simulink model "DDDR"  (R2020a)
settings: Solver=FixedStepAuto  StartTime=0.0  StopTime=50.0  FixedStep=1e-3  RelTol=1e-3  EnableMultiTasking=on
undefined symbols (not defined in the file): A0, A1, A3, D0, D1, D10, D11, D12, D13, D2, D3, D4, D5, D6, D7, D8, D9, PTA0, PTA1, PTA2, PTB11, PTB2, PTB23, PTB3, PTB9, PTC16, PTC17, PTC2, PTC3, PTC4, PTD0, PTD1, PTD2, PTD3
libraries: etargetslib x44, frdmk64flib x22, dspstat3 x1
(part 1 of 2)
settings Model: ExtModeTrigDuration=5  Creator=safanaal-emara  LastModifiedBy=prana
settings OptimizationCC: EnhancedBackFolding=on  PassReuseOutputArgsAs=Individual arguments  ZeroExternalMemoryAtStartup=off  ZeroInternalMemoryAtStartup=off  MaxStackSize=64  OptimizeBlockOrder=speed  DifferentSizesBufferReuse=on  OptimizationCustomize=off  EfficientTunableParamExpr=on
settings DebuggingCC: ParameterTunabilityLossMsg=error
settings HardwareCC: ProdBitPerPointer=32  ProdBitPerSizeT=32  ProdBitPerPtrDiffT=32  ProdLargestAtomicInteger=Long  ProdLargestAtomicFloat=Double  ProdWordSize=32  ProdHWDeviceType=ARM Compatible->ARM Cortex
settings SFSimCC: MATLABDynamicMemAlloc=off
settings RTWCC: SystemTargetFile=ert.tlc  HardwareBoard=NXP FRDM-K64F  TemplateMakefile=ert_default_tmf  Toolchain=GNU Tools for ARM Embedded Processors
settings CodeAppCC: ForceParamTrailComments=on  IgnoreCustomStorageClasses=off  OperatorAnnotations=on  SimulinkDataObjDesc=on  SFDataObjDesc=on  InsertBlockDesc=on
settings ERTTargetCC: SupportVariableSizeSignals=on

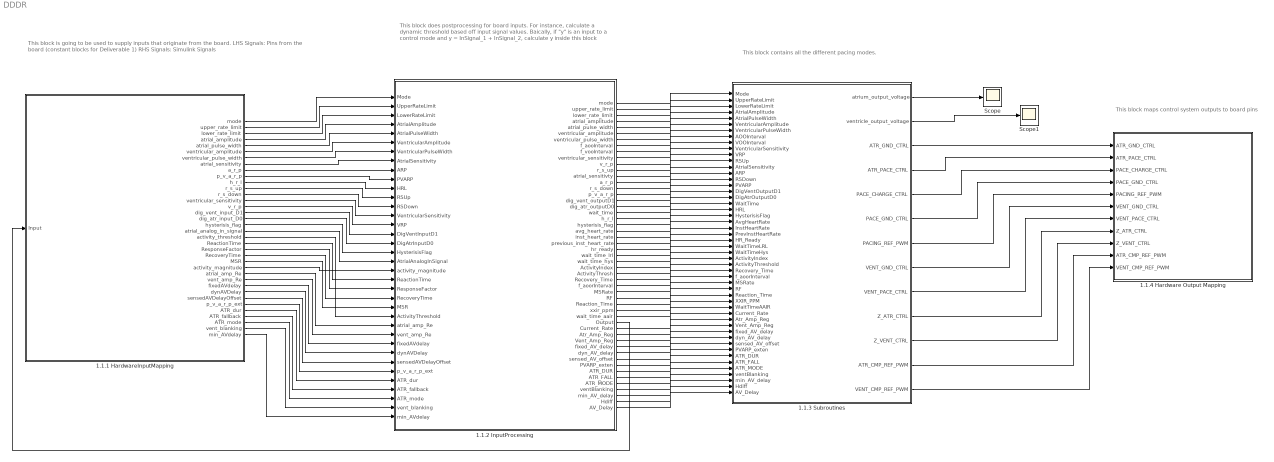
== system DDDR ==
  note: This block is going to be used to supply inputs that originate from the board.
      | LHS Signals: Pins from the board (constant blocks for Deliverable 1)
      | RHS Signals: Simulink Signals
  note: This block contains all the different pacing modes.
  note: This block does postprocessing for board inputs.
      | For instance, calculate a dynamic threshold based off input signal values.
      | Baically, if "y" is an input to a control mode and y = InSignal_1 + InSignal_2,
      | calculate y inside this block
  note: This block maps control system outputs to board pins
  1.1.1 HardwareInputMapping : Subsystem
  1.1.2 InputProcessing : Subsystem
  1.1.3 Subroutines : Subsystem
  1.1.4 Hardware Output Mapping : Subsystem
  Scope : Scope
  Scope1 : Scope
  wires:
  1.1.1 HardwareInputMapping/23(RecoveryTime) -> 1.1.2 InputProcessing/23(RecoveryTime)
  1.1.2 InputProcessing/30(Recovery_Time) -> 1.1.3 Subroutines/30(Recovery_Time)
  1.1.3 Subroutines/5(PACE_CHARGE_CTRL) -> 1.1.4 Hardware Output Mapping/3(PACE_CHARGE_CTRL)
  1.1.2 InputProcessing/31(f_aoorInterval) -> 1.1.3 Subroutines/31(f_aoorInterval)
  1.1.2 InputProcessing/19(wait_time) -> 1.1.3 Subroutines/19(WaitTime)
  1.1.2 InputProcessing/29(ActivityThresh) -> 1.1.3 Subroutines/29(ActivityThreshold)
  1.1.1 HardwareInputMapping/20(activity_threshold) -> 1.1.2 InputProcessing/25(ActivityThreshold)
  1.1.3 Subroutines/8(VENT_GND_CTRL) -> 1.1.4 Hardware Output Mapping/6(VENT_GND_CTRL)
  1.1.1 HardwareInputMapping/5(atrial_pulse_width) -> 1.1.2 InputProcessing/5(AtrialPulseWidth)
  1.1.3 Subroutines/12(ATR_CMP_REF_PWM) -> 1.1.4 Hardware Output Mapping/10(ATR_CMP_REF_PWM)
  1.1.3 Subroutines/13(VENT_CMP_REF_PWM) -> 1.1.4 Hardware Output Mapping/11(VENT_CMP_REF_PWM)
  1.1.2 InputProcessing/28(ActivityIndex) -> 1.1.3 Subroutines/28(ActivityIndex)
  1.1.3 Subroutines/6(PACE_GND_CTRL) -> 1.1.4 Hardware Output Mapping/4(PACE_GND_CTRL)
  1.1.2 InputProcessing/15(r_s_down) -> 1.1.3 Subroutines/15(RSDown)
  1.1.1 HardwareInputMapping/16(dig_vent_input_D1) -> 1.1.2 InputProcessing/16(DigVentInputD1)
  1.1.2 InputProcessing/32(MSRate) -> 1.1.3 Subroutines/32(MSRate)
  1.1.1 HardwareInputMapping/24(MSR) -> 1.1.2 InputProcessing/24(MSR)
  1.1.3 Subroutines/3(ATR_GND_CTRL) -> 1.1.4 Hardware Output Mapping/1(ATR_GND_CTRL)
  1.1.2 InputProcessing/26(wait_time_lrl) -> 1.1.3 Subroutines/26(WaitTimeLRL)
  1.1.2 InputProcessing/16(p_v_a_r_p) -> 1.1.3 Subroutines/16(PVARP)
  1.1.3 Subroutines/7(PACING_REF_PWM) -> 1.1.4 Hardware Output Mapping/5(PACING_REF_PWM)
  1.1.2 InputProcessing/27(wait_time_hys) -> 1.1.3 Subroutines/27(WaitTimeHys)
  1.1.2 InputProcessing/13(atrial_sensitivty) -> 1.1.3 Subroutines/13(AtrialSensitivity)
  1.1.2 InputProcessing/14(a_r_p) -> 1.1.3 Subroutines/14(ARP)
  1.1.1 HardwareInputMapping/3(lower_rate_limit) -> 1.1.2 InputProcessing/3(LowerRateLimit)
  1.1.2 InputProcessing/25(hr_ready) -> 1.1.3 Subroutines/25(HR_Ready)
  1.1.1 HardwareInputMapping/19(atrial_analog_in_signal) -> 1.1.2 InputProcessing/19(AtrialAnalogInSignal)
  1.1.2 InputProcessing/20(h_r_l) -> 1.1.3 Subroutines/20(HRL)
  1.1.2 InputProcessing/23(inst_heart_rate) -> 1.1.3 Subroutines/23(InstHeartRate)
  1.1.2 InputProcessing/10(ventricular_sensitivity) -> 1.1.3 Subroutines/10(VentricularSensitivity)
  1.1.2 InputProcessing/22(avg_heart_rate) -> 1.1.3 Subroutines/22(AvgHeartRate)
  1.1.3 Subroutines/11(Z_VENT_CTRL) -> 1.1.4 Hardware Output Mapping/9(Z_VENT_CTRL)
  1.1.3 Subroutines/10(Z_ATR_CTRL) -> 1.1.4 Hardware Output Mapping/8(Z_ATR_CTRL)
  1.1.3 Subroutines/9(VENT_PACE_CTRL) -> 1.1.4 Hardware Output Mapping/7(VENT_PACE_CTRL)
  1.1.1 HardwareInputMapping/14(ventricular_sensitivity) -> 1.1.2 InputProcessing/14(VentricularSensitivity)
  1.1.2 InputProcessing/34(Reaction_Time) -> 1.1.3 Subroutines/34(Reaction_Time)
  1.1.3 Subroutines/4(ATR_PACE_CTRL) -> 1.1.4 Hardware Output Mapping/2(ATR_PACE_CTRL)
  1.1.2 InputProcessing/17(dig_vent_outputD1) -> 1.1.3 Subroutines/17(DigVentOutputD1)
  1.1.1 HardwareInputMapping/11(h_r_l) -> 1.1.2 InputProcessing/11(HRL)
  1.1.1 HardwareInputMapping/7(ventricular_pulse_width) -> 1.1.2 InputProcessing/7(VentricularPulseWidth)
  1.1.1 HardwareInputMapping/10(p_v_a_r_p) -> 1.1.2 InputProcessing/10(PVARP)
  1.1.2 InputProcessing/11(v_r_p) -> 1.1.3 Subroutines/11(VRP)
  1.1.1 HardwareInputMapping/13(r_s_down) -> 1.1.2 InputProcessing/13(RSDown)
  1.1.2 InputProcessing/5(atrial_pulse_width) -> 1.1.3 Subroutines/5(AtrialPulseWidth)
  1.1.1 HardwareInputMapping/9(a_r_p) -> 1.1.2 InputProcessing/9(ARP)
  1.1.2 InputProcessing/36(wait_time_aair) -> 1.1.3 Subroutines/36(WaitTimeAAIR)
  1.1.2 InputProcessing/21(hysterisis_flag) -> 1.1.3 Subroutines/21(HysterisisFlag)
  1.1.1 HardwareInputMapping/17(dig_atr_input_D0) -> 1.1.2 InputProcessing/17(DigAtrInputD0)
  1.1.2 InputProcessing/7(ventricular_pulse_width) -> 1.1.3 Subroutines/7(VentricularPulseWidth)
  1.1.1 HardwareInputMapping/8(atrial_sensitivity) -> 1.1.2 InputProcessing/8(AtrialSensitivity)
  1.1.1 HardwareInputMapping/6(ventricular_amplitude) -> 1.1.2 InputProcessing/6(VentricularAmplitude)
  1.1.2 InputProcessing/33(RF) -> 1.1.3 Subroutines/33(RF)
  1.1.2 InputProcessing/3(lower_rate_limit) -> 1.1.3 Subroutines/3(LowerRateLimit)
  1.1.2 InputProcessing/24(previous_inst_heart_rate) -> 1.1.3 Subroutines/24(PrevInstHeartRate)
  1.1.2 InputProcessing/12(r_s_up) -> 1.1.3 Subroutines/12(RSUp)
  1.1.1 HardwareInputMapping/4(atrial_amplitude) -> 1.1.2 InputProcessing/4(AtrialAmplitude)
  1.1.2 InputProcessing/18(dig_atr_outputD0) -> 1.1.3 Subroutines/18(DigAtrOutputD0)
  1.1.3 Subroutines/2(ventricle_output_voltage) -> Scope1/1
  1.1.1 HardwareInputMapping/1(mode) -> 1.1.2 InputProcessing/1(Mode)
  1.1.3 Subroutines/1(atrium_output_voltage) -> Scope/1
  1.1.1 HardwareInputMapping/21(ReactionTime) -> 1.1.2 InputProcessing/21(ReactionTime)
  1.1.2 InputProcessing/4(atrial_amplitude) -> 1.1.3 Subroutines/4(AtrialAmplitude)
  1.1.2 InputProcessing/6(ventricular_amplitude) -> 1.1.3 Subroutines/6(VentricularAmplitude)
  1.1.1 HardwareInputMapping/18(hysterisis_flag) -> 1.1.2 InputProcessing/18(HysterisisFlag)
  1.1.2 InputProcessing/9(f_vooInterval) -> 1.1.3 Subroutines/9(VOOInterval)
  1.1.2 InputProcessing/1(mode) -> 1.1.3 Subroutines/1(Mode)
  1.1.1 HardwareInputMapping/22(ResponseFactor) -> 1.1.2 InputProcessing/22(ResponseFactor)
  1.1.1 HardwareInputMapping/15(v_r_p) -> 1.1.2 InputProcessing/15(VRP)
  1.1.1 HardwareInputMapping/2(upper_rate_limit) -> 1.1.2 InputProcessing/2(UpperRateLimit)
  1.1.2 InputProcessing/2(upper_rate_limit) -> 1.1.3 Subroutines/2(UpperRateLimit)
  1.1.1 HardwareInputMapping/12(r_s_up) -> 1.1.2 InputProcessing/12(RSUp)
  1.1.2 InputProcessing/8(f_aooInterval) -> 1.1.3 Subroutines/8(AOOInterval)
  1.1.2 InputProcessing/35(xxir_ppm) -> 1.1.3 Subroutines/35(XXIR_PPM)
  1.1.1 HardwareInputMapping/25(activity_magnitude) -> 1.1.2 InputProcessing/20(activity_magnitude)
  1.1.2 InputProcessing/37(Output) -> 1.1.1 HardwareInputMapping/1(Input)
  1.1.2 InputProcessing/38(Current_Rate) -> 1.1.3 Subroutines/37(Current_Rate)
  1.1.1 HardwareInputMapping/26(atrial_amp_Re) -> 1.1.2 InputProcessing/26(atrial_amp_Re)
  1.1.1 HardwareInputMapping/27(vent_amp_Re) -> 1.1.2 InputProcessing/27(vent_amp_Re)
  1.1.2 InputProcessing/39(Atr_Amp_Reg) -> 1.1.3 Subroutines/38(Atr_Amp_Reg)
  1.1.2 InputProcessing/40(Vent_Amp_Reg) -> 1.1.3 Subroutines/39(Vent_Amp_Reg)
  1.1.1 HardwareInputMapping/28(fixedAVdelay) -> 1.1.2 InputProcessing/28(fixedAVdelay)
  1.1.1 HardwareInputMapping/29(dynAVDelay) -> 1.1.2 InputProcessing/29(dynAVDelay)
  1.1.1 HardwareInputMapping/30(sensedAVDelayOffset) -> 1.1.2 InputProcessing/30(sensedAVDelayOffset)
  1.1.1 HardwareInputMapping/31(p_v_a_r_p_ext) -> 1.1.2 InputProcessing/31(p_v_a_r_p_ext)
  1.1.1 HardwareInputMapping/32(ATR_dur) -> 1.1.2 InputProcessing/32(ATR_dur)
  1.1.1 HardwareInputMapping/33(ATR_fallback) -> 1.1.2 InputProcessing/33(ATR_fallback)
  1.1.1 HardwareInputMapping/34(ATR_mode) -> 1.1.2 InputProcessing/34(ATR_mode)
  1.1.1 HardwareInputMapping/35(vent_blanking) -> 1.1.2 InputProcessing/35(vent_blanking)
  1.1.1 HardwareInputMapping/36(min_AVdelay) -> 1.1.2 InputProcessing/36(min_AVdelay)
  1.1.2 InputProcessing/41(fixed_AV_delay) -> 1.1.3 Subroutines/40(fixed_AV_delay)
  1.1.2 InputProcessing/42(dyn_AV_delay) -> 1.1.3 Subroutines/41(dyn_AV_delay)
  1.1.2 InputProcessing/43(sensed_AV_offset) -> 1.1.3 Subroutines/42(sensed_AV_offset)
  1.1.2 InputProcessing/44(PVARP_exten) -> 1.1.3 Subroutines/43(PVARP_exten)
  1.1.2 InputProcessing/45(ATR_DUR) -> 1.1.3 Subroutines/44(ATR_DUR)
  1.1.2 InputProcessing/46(ATR_FALL) -> 1.1.3 Subroutines/45(ATR_FALL)
  1.1.2 InputProcessing/47(ATR_MODE) -> 1.1.3 Subroutines/46(ATR_MODE)
  1.1.2 InputProcessing/48(ventBlanking) -> 1.1.3 Subroutines/47(ventBlanking)
  1.1.2 InputProcessing/49(min_AV_delay) -> 1.1.3 Subroutines/48(min_AV_delay)
  1.1.2 InputProcessing/50(Hdiff) -> 1.1.3 Subroutines/49(Hdiff)
  1.1.2 InputProcessing/51(AV_Delay) -> 1.1.3 Subroutines/50(AV_Delay)

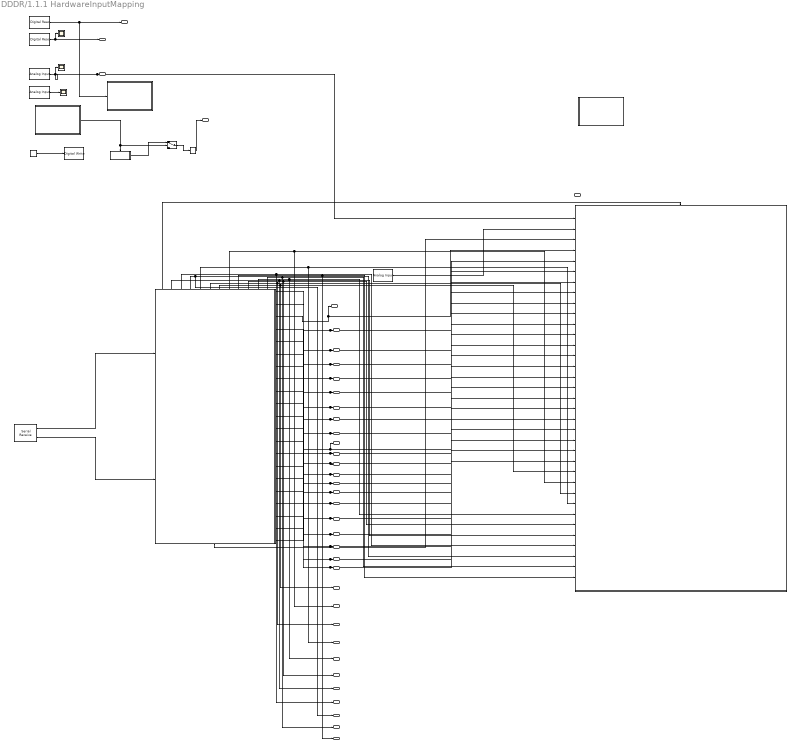
== system DDDR/1.1.1 HardwareInputMapping ==
  note: Technically should be in 1.1.2, but remains here for sake of testing ease
  note: Hardware Abstraction
  Input : Inport  OutDataTypeStr=uint32
  ATR_CMP_DETECT : frdmk64flib/Digital Read  Whichpin=PTC16 (D0)  SampleTime=0.001
  Analog Input : frdmk64flib/Analog Input  Whichpin=PTB2 (A0)  SampleTime=0.001
  Analog Input1 : frdmk64flib/Analog Input  Whichpin=PTB11 (A3)  SampleTime=0.001
  Analog Input4 : frdmk64flib/Analog Input  Whichpin=PTB3 (A1)  SampleTime=0.001
  Chart1 : Stateflow chart  TreatAsAtomicUnit=on
      settings: PortSchema="{\"entries\":[{\"content\":{\"sides\":[{\"content\":{\"connectorIds\":[\"In1\",\"In2\"]},\"type\":\"ConnectorPlacement.EquallySpacedRectSide\",\"uuid\":\"4b4e7b92-92d9-42ab-8219-d0bebd29739c\"},{\"content\":{\"connectorIds\":[\"Out2\",\"Out3\",\"Out4\",\"Out5\",\"Out6\",\"Out7\",\"Out8\",\"Out9\",\"Out10\",\"Out11\",\"Out12\",\"Out13\",\"Out14\",\"Out15\",\"Out16\",\"Out17\",\"Out18\",\"Out19\",\"Out20\",\"Out21\",\"Out22\"],\"side\":\"RIGHT\"},\"type\":\"ConnectorPlacement.EquallySpacedRectSide\",\"uuid\":\"63818af1-55be-4bb8-9c31-e72eb1b14a30\"},{\"content\":{\"connectorIds\":[\"Out23\",\"Out24\",\"Out25\",\"Out26\",\"Out27\",\"Out28\",\"Out29\",\"Out30\",\"Out31\",\"Out32\",\"Out33\",\"Out34\"],\"side\":\"TOP\"},\"type\":\"ConnectorPlacement.EquallySpacedRectSide\",\"uuid\":\"fba88a00-7af7-4cc1-9c88-2f6823948803\"},{\"content\":{\"connectorIds\":[\"Out1\"],\"side\":\"BOTTOM\"},\"type\":\"ConnectorPlacement.EquallySpacedRectSide\",\"uuid\":\"45b0438b-424b-4dc6-9f15-00cd0d7c78e5\"}]},\"type\":\"ConnectorPlacement.EquallySpacedConnector\",\"uuid\":\"faeef76d-5f3a-4672-ae10-d5c9531e9562\"}],\"packageUris\":[\"http://schema.mathworks.com/mf0/Connector/19700101\"],\"version\":\"1.0\"}"
  Constant15 : Constant  Value=true  OutDataTypeStr=boolean
  Digital Write1 : frdmk64flib/Digital Write  Whichpin=PTD1 (D13)
  HeartChamberPulseDetection : Stateflow chart  TreatAsAtomicUnit=on
  HeartChamberPulseDetection2 : Stateflow chart  TreatAsAtomicUnit=on
  HeartChamberPulseDetection3 : Stateflow chart  TreatAsAtomicUnit=on
  Memory : Memory
  Scope : Scope
  Scope1 : Scope
  Scope2 : Scope
  Serial Receive : frdmk64flib/Serial Receive  SCIModule=0  Baudrate=uint32(9600)  Parity=None  StopBits=1  HardwareFlowControl=None  ByteOrder=LittleEndian  DataType=uint8  DataLength=125  BlockingMode=off  OutputStatus=on  SampleTime=-1
  Subsystem1 : Subsystem
  Switch : Switch  Criteria=u2 > Threshold
  Triggered Subsystem : Subsystem  TreatAsAtomicUnit=on
  VENT_CMP_DETECT : frdmk64flib/Digital Read  Whichpin=PTC17 (D1)  SampleTime=0.001
  mode : Outport  OutDataTypeStr=uint32
  upper_rate_limit : Outport  Port=2
  lower_rate_limit : Outport  Port=3  OutDataTypeStr=uint32
  atrial_amplitude : Outport  Port=4
  atrial_pulse_width : Outport  Port=5
  ventricular_amplitude : Outport  Port=6
  ventricular_pulse_width : Outport  Port=7
  atrial_sensitivity : Outport  Port=8
  a_r_p : Outport  Port=9
  p_v_a_r_p : Outport  Port=10
  h_r_l : Outport  Port=11
  r_s_up : Outport  Port=12
  r_s_down : Outport  Port=13
  ventricular_sensitivity : Outport  Port=14
  v_r_p : Outport  Port=15
  dig_vent_input_D1 : Outport  Port=16
  dig_atr_input_D0 : Outport  Port=17
  hysterisis_flag : Outport  Port=18
  atrial_analog_in_signal : Outport  Port=19
  activity_threshold : Outport  Port=20
  ReactionTime : Outport  Port=21
  ResponseFactor : Outport  Port=22
  RecoveryTime : Outport  Port=23
  MSR : Outport  Port=24
  activity_magnitude : Outport  Port=25
  atrial_amp_Re : Outport  Port=26
  vent_amp_Re : Outport  Port=27
  fixedAVdelay : Outport  Port=28
  dynAVDelay : Outport  Port=29
  sensedAVDelayOffset : Outport  Port=30
  p_v_a_r_p_ext : Outport  Port=31
  ATR_dur : Outport  Port=32
  ATR_fallback : Outport  Port=33
  ATR_mode : Outport  Port=34
  vent_blanking : Outport  Port=35
  min_AVdelay : Outport  Port=36
  wires:
  ATR_CMP_DETECT/1 -> Scope/1, dig_atr_input_D0/1
  Constant15/1 -> Digital Write1/1
  VENT_CMP_DETECT/1 -> dig_vent_input_D1/1, HeartChamberPulseDetection/1(in_voltage)
  Chart1/4(Mode) -> Subsystem1/4(Mode), mode/1
  Chart1/2(MSR) -> Subsystem1/24(m_s_r), MSR/1
  Chart1/3(ReactionTime) -> Subsystem1/21(Reaction_time), ReactionTime/1
  Chart1/5(RecoveryTime) -> Subsystem1/23(recovery_time), RecoveryTime/1
  Chart1/6(ResponseFactor) -> Subsystem1/22(Response_factor), ResponseFactor/1
  Chart1/7(a_r_p) -> Subsystem1/12(ARP), a_r_p/1
  Chart1/9(atrial_amplitude) -> Subsystem1/7(AtrialAmplitude), atrial_amplitude/1
  Chart1/10(atrial_pulse_width) -> Subsystem1/8(AtrialPulseWidth), atrial_pulse_width/1
  Chart1/11(atrial_sensitivity) -> Subsystem1/11(AtrialSensitivity), atrial_sensitivity/1
  Chart1/12(h_r_l) -> Subsystem1/14(HRL), h_r_l/1
  Chart1/13(hysterisis_flag) -> Subsystem1/18(HysterisisFlag1), hysterisis_flag/1
  Chart1/14(lower_rate_limit) -> Subsystem1/6(LowerRateLimit), lower_rate_limit/1
  Chart1/15(p_v_a_r_p) -> Subsystem1/13(PVARP), p_v_a_r_p/1
  Chart1/16(r_s_down) -> Subsystem1/16(RSDown), r_s_down/1
  Chart1/17(r_s_up) -> Subsystem1/15(RSUp), r_s_up/1
  Chart1/18(upper_rate_limit) -> Subsystem1/5(UpperRateLimit), upper_rate_limit/1
  Chart1/19(v_r_p) -> Subsystem1/19(VRP), v_r_p/1
  Chart1/20(ventricular_amplitude) -> Subsystem1/9(VentricularAmplitude), ventricular_amplitude/1
  Chart1/21(ventricular_pulse_width) -> Subsystem1/10(VentricularPulseWidth), ventricular_pulse_width/1
  Chart1/22(ventricular_sensitivity) -> Subsystem1/17(VentricularSensitivity), ventricular_sensitivity/1
  Serial Receive/1 -> Chart1/1(rx_data)
  Serial Receive/2 -> Chart1/2(status)
  Chart1/23(MSG_trigger) -> Subsystem1/Trigger
  Chart1/8(activity_threshold) -> Subsystem1/20(Activity_threshold), activity_threshold/1
  HeartChamberPulseDetection3/1(LED_STATE) -> Triggered Subsystem/Trigger, Switch/2
  Switch/1 -> Memory/1
  Memory/1 -> activity_magnitude/1
  Triggered Subsystem/1(activity_magnitude) -> Switch/1
  Chart1/1(MSG_ident) -> Subsystem1/3(MSG_ident)
  Analog Input4/1 -> Subsystem1/2(Vent_signal)
  Analog Input1/1 -> Scope2/1
  Analog Input/1 -> Subsystem1/1(Atrial_signal), atrial_analog_in_signal/1, Scope1/1
  Chart1/29(atrial_amplitude_Re) -> atrial_amp_Re/1, Subsystem1/25(atr_amp_re)
  Chart1/30(ventricular_amplitude_Re) -> vent_amp_Re/1, Subsystem1/26(vent_amp_re)
  Chart1/28(Fixed_AV_delay) -> fixedAVdelay/1, Subsystem1/27(fixed_AV_delay)
  Chart1/27(Dynamic_AV_delay) -> dynAVDelay/1, Subsystem1/28(dynamic_AV_delay)
  Chart1/33(sensed_AV_delay_offset) -> sensedAVDelayOffset/1, Subsystem1/29(sensed_AV_delay_offset)
  Chart1/32(p_v_a_r_p_ext) -> p_v_a_r_p_ext/1, Subsystem1/30(pvarp_ext)
  Chart1/24(ATR_dur) -> ATR_dur/1, Subsystem1/31(ATR_dur)
  Chart1/25(ATR_fallback_time) -> ATR_fallback/1, Subsystem1/32(ATR_fallback)
  Chart1/26(ATR_mode) -> ATR_mode/1, Subsystem1/33(ATR_mode)
  Chart1/34(vent_blanking) -> vent_blanking/1, Subsystem1/34(vent_blanking)
  Chart1/31(min_AV_delay) -> min_AVdelay/1, Subsystem1/35(min_dyn_AV_delay)

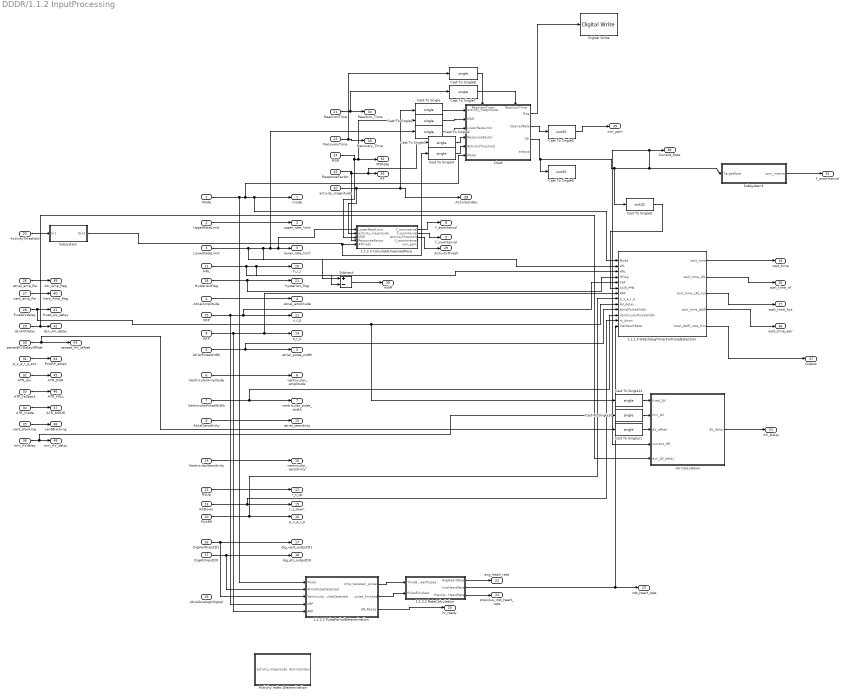
== system DDDR/1.1.2 InputProcessing ==
  Mode : Inport
  UpperRateLimit : Inport  Port=2
  LowerRateLimit : Inport  Port=3  OutDataTypeStr=uint32
  AtrialAmplitude : Inport  Port=4
  AtrialPulseWidth : Inport  Port=5
  VentricularAmplitude : Inport  Port=6
  VentricularPulseWidth : Inport  Port=7
  AtrialSensitivity : Inport  Port=8
  ARP : Inport  Port=9
  PVARP : Inport  Port=10
  HRL : Inport  Port=11
  RSUp : Inport  Port=12
  RSDown : Inport  Port=13
  VentricularSensitivity : Inport  Port=14
  VRP : Inport  Port=15
  DigVentInputD1 : Inport  Port=16
  DigAtrInputD0 : Inport  Port=17
  HysterisisFlag : Inport  Port=18
  AtrialAnalogInSignal : Inport  Port=19
  activity_magnitude : Inport  Port=20
  ReactionTime : Inport  Port=21
  ResponseFactor : Inport  Port=22
  RecoveryTime : Inport  Port=23
  MSR : Inport  Port=24
  ActivityThreshold : Inport  Port=25
  atrial_amp_Re : Inport  Port=26
  vent_amp_Re : Inport  Port=27
  fixedAVdelay : Inport  Port=28
  dynAVDelay : Inport  Port=29
  sensedAVDelayOffset : Inport  Port=30
  p_v_a_r_p_ext : Inport  Port=31
  ATR_dur : Inport  Port=32
  ATR_fallback : Inport  Port=33
  ATR_mode : Inport  Port=34
  vent_blanking : Inport  Port=35
  min_AVdelay : Inport  Port=36
  1.1.2.1 PulsePeriodDetermination : Stateflow chart  TreatAsAtomicUnit=on
  1.1.2.2 RateCalculation : Subsystem
  1.1.2.3 WatchdogTimerForPulseDetection : Stateflow chart  TreatAsAtomicUnit=on
      settings: PortSchema="{\"entries\":[{\"content\":{\"sides\":[{\"content\":{\"connectorIds\":[\"In2\",\"In4\",\"In3\",\"In1\",\"In8\",\"In10\",\"In11\",\"In12\",\"In13\",\"In5\",\"In6\",\"In9\",\"In7\"]},\"type\":\"ConnectorPlacement.EquallySpacedRectSide\",\"uuid\":\"bdcd44c7-b2d4-4456-b1dc-ebe8b4250225\"},{\"content\":{\"connectorIds\":[\"Out1\",\"Out2\",\"Out3\",\"Out4\",\"Out5\"],\"side\":\"RIGHT\"},\"type\":\"ConnectorPlacement.EquallySpacedRectSide\",\"uuid\":\"3cd61675-91fc-4dc9-8435-a65c8d2417e3\"},{\"content\":{\"connectorIds\":[],\"side\":\"TOP\"},\"type\":\"ConnectorPlacement.EquallySpacedRectSide\",\"uuid\":\"27150ff9-b670-45e1-a88f-5aa1ecaf40ee\"}]},\"type\":\"ConnectorPlacement.EquallySpacedConnector\",\"uuid\":\"8013b024-43b4-4f43-9604-3ddd237ba5b0\"}],\"packageUris\":[\"http://schema.mathworks.com/mf0/Connector/19700101\"],\"version\":\"1.0\"}"
  1.1.2.4 CalculateUnsensedPace : Subsystem
  AV Calculation : Stateflow chart  TreatAsAtomicUnit=on
  Activity Index Determination : Stateflow chart  TreatAsAtomicUnit=on
  Cast To Single{,1..4,7..8,10..12} (10 alike) : DataTypeConversion  OutDataTypeStr=single
  Cast To Single5 : DataTypeConversion  OutDataTypeStr=uint32
  Cast To Single6 : DataTypeConversion  OutDataTypeStr=uint32
  Cast To Single9 : DataTypeConversion  OutDataTypeStr=uint32
  Chart : Stateflow chart  TreatAsAtomicUnit=on
      settings: PortSchema="{\"entries\":[{\"content\":{\"sides\":[{\"content\":{\"connectorIds\":[\"In3\",\"In4\",\"In5\",\"In6\",\"In7\",\"In8\"]},\"type\":\"ConnectorPlacement.EquallySpacedRectSide\",\"uuid\":\"2448e127-c765-4c5f-8f36-5c1cc0db25c5\"},{\"content\":{\"connectorIds\":[\"Out1\",\"Out2\",\"Out3\",\"Out4\"],\"side\":\"RIGHT\"},\"type\":\"ConnectorPlacement.EquallySpacedRectSide\",\"uuid\":\"7735dab6-aae1-403a-9bfd-50f09b6b5fda\"},{\"content\":{\"connectorIds\":[\"In1\",\"In2\"],\"side\":\"TOP\"},\"type\":\"ConnectorPlacement.EquallySpacedRectSide\",\"uuid\":\"b73b27d3-29c6-41fa-95b7-891e2a296021\"}]},\"type\":\"ConnectorPlacement.EquallySpacedConnector\",\"uuid\":\"e62d7f02-cd80-41b6-aa16-da75d3dcce48\"}],\"packageUris\":[\"http://schema.mathworks.com/mf0/Connector/19700101\"],\"version\":\"1.0\"}"
  Digital Write : frdmk64flib/Digital Write  Whichpin=GREEN_LED
  Subsystem : Subsystem
  Subsystem1 : Subsystem
  Subtract : Sum  Inputs=+-
  mode : Outport  OutDataTypeStr=uint32
  upper_rate_limit : Outport  Port=2
  lower_rate_limit : Outport  Port=3
  atrial_amplitude : Outport  Port=4
  atrial_pulse_width : Outport  Port=5
  ventricular_amplitude : Outport  Port=6
  ventricular_pulse_width : Outport  Port=7
  f_aooInterval : Outport  Port=8
  f_vooInterval : Outport  Port=9
  ventricular_sensitivity : Outport  Port=10
  v_r_p : Outport  Port=11
  r_s_up : Outport  Port=12
  atrial_sensitivty : Outport  Port=13
  a_r_p : Outport  Port=14
  r_s_down : Outport  Port=15
  p_v_a_r_p : Outport  Port=16
  dig_vent_outputD1 : Outport  Port=17
  dig_atr_outputD0 : Outport  Port=18
  wait_time : Outport  Port=19
  h_r_l : Outport  Port=20
  hysterisis_flag : Outport  Port=21
  avg_heart_rate : Outport  Port=22
  inst_heart_rate : Outport  Port=23
  previous_inst_heart_rate : Outport  Port=24
  hr_ready : Outport  Port=25
  wait_time_lrl : Outport  Port=26
  wait_time_hys : Outport  Port=27
  ActivityIndex : Outport  Port=28
  ActivityThresh : Outport  Port=29
  Recovery_Time : Outport  Port=30
  f_aoorInterval : Outport  Port=31  OutDataTypeStr=uint32
  MSRate : Outport  Port=32
  RF : Outport  Port=33
  Reaction_Time : Outport  Port=34
  xxir_ppm : Outport  Port=35
  wait_time_aair : Outport  Port=36
  Output : Outport  Port=37
  Current_Rate : Outport  Port=38
  Atr_Amp_Reg : Outport  Port=39
  Vent_Amp_Reg : Outport  Port=40
  fixed_AV_delay : Outport  Port=41
  dyn_AV_delay : Outport  Port=42
  sensed_AV_offset : Outport  Port=43
  PVARP_exten : Outport  Port=44
  ATR_DUR : Outport  Port=45
  ATR_FALL : Outport  Port=46
  ATR_MODE : Outport  Port=47
  ventBlanking : Outport  Port=48
  min_AV_delay : Outport  Port=49
  Hdiff : Outport  Port=50
  AV_Delay : Outport  Port=51  OutDataTypeStr=single
  wires:
  Mode/1 -> 1.1.2.1 PulsePeriodDetermination/1(Mode), Chart/8(Mode), 1.1.2.3 WatchdogTimerForPulseDetection/2(Mode), mode/1
  UpperRateLimit/1 -> upper_rate_limit/1
  LowerRateLimit/1 -> Subtract/1, Cast To Single2/1, 1.1.2.4 CalculateUnsensedPace/1(LowerRateLimit), lower_rate_limit/1, 1.1.2.3 WatchdogTimerForPulseDetection/4(LRL)
  AtrialAmplitude/1 -> atrial_amplitude/1
  AtrialPulseWidth/1 -> 1.1.2.3 WatchdogTimerForPulseDetection/5(AtrialPulseWidth), atrial_pulse_width/1
  VentricularAmplitude/1 -> ventricular_amplitude/1
  VentricularPulseWidth/1 -> 1.1.2.3 WatchdogTimerForPulseDetection/6(VentricularPulseWidth), ventricular_pulse_width/1
  1.1.2.4 CalculateUnsensedPace/1(f_aooInterval) -> f_aooInterval/1
  1.1.2.4 CalculateUnsensedPace/2(f_vooInterval) -> f_vooInterval/1
  VentricularSensitivity/1 -> ventricular_sensitivity/1
  VRP/1 -> 1.1.2.1 PulsePeriodDetermination/4(VRP), 1.1.2.3 WatchdogTimerForPulseDetection/8(VRP), v_r_p/1
  RSUp/1 -> r_s_up/1
  AtrialSensitivity/1 -> atrial_sensitivty/1
  ARP/1 -> 1.1.2.1 PulsePeriodDetermination/5(ARP), 1.1.2.3 WatchdogTimerForPulseDetection/11(ARP), a_r_p/1
  RSDown/1 -> 1.1.2.3 WatchdogTimerForPulseDetection/9(rs_down), r_s_down/1
  PVARP/1 -> 1.1.2.3 WatchdogTimerForPulseDetection/12(p_v_a_r_p), p_v_a_r_p/1
  HRL/1 -> Subtract/2, 1.1.2.3 WatchdogTimerForPulseDetection/3(HRL), h_r_l/1
  DigVentInputD1/1 -> 1.1.2.1 PulsePeriodDetermination/3(VentricularPulseDetected), dig_vent_outputD1/1
  DigAtrInputD0/1 -> 1.1.2.1 PulsePeriodDetermination/2(AtrialPulseDetected), dig_atr_outputD0/1
  HysterisisFlag/1 -> 1.1.2.3 WatchdogTimerForPulseDetection/1(HFlag), hysterisis_flag/1
  1.1.2.3 WatchdogTimerForPulseDetection/1(wait_time) -> wait_time/1
  1.1.2.1 PulsePeriodDetermination/1(time_between_pulses) -> 1.1.2.2 RateCalculation/1(TimeBetweenPulses)
  1.1.2.2 RateCalculation/1(AvgHeartRate) -> avg_heart_rate/1
  1.1.2.2 RateCalculation/3(PrevInstHeartRate) -> previous_inst_heart_rate/1
  1.1.2.2 RateCalculation/2(InstHeartRate) -> 1.1.2.3 WatchdogTimerForPulseDetection/7(InstHeartRate), inst_heart_rate/1
  1.1.2.1 PulsePeriodDetermination/3(HR_Ready) -> hr_ready/1
  1.1.2.1 PulsePeriodDetermination/2(pulse_finished) -> 1.1.2.2 RateCalculation/2(PulseFinished)
  1.1.2.3 WatchdogTimerForPulseDetection/2(wait_time_LRL) -> wait_time_lrl/1
  1.1.2.3 WatchdogTimerForPulseDetection/3(wait_time_LRL_hys) -> wait_time_hys/1
  activity_magnitude/1 -> 1.1.2.4 CalculateUnsensedPace/2(activity_magnitude), Cast To Single/1, ActivityIndex/1
  ActivityThreshold/1 -> Subsystem/1(In1)
  1.1.2.4 CalculateUnsensedPace/3(ActivityThreshold) -> ActivityThresh/1
  MSR/1 -> 1.1.2.4 CalculateUnsensedPace/3(MSR), MSRate/1, Cast To Single1/1
  ResponseFactor/1 -> Cast To Single3/1, RF/1, 1.1.2.4 CalculateUnsensedPace/4(ResponseFactor)
  RecoveryTime/1 -> Cast To Single8/1, Recovery_Time/1
  1.1.2.3 WatchdogTimerForPulseDetection/4(wait_time_AAIR) -> wait_time_aair/1
  Chart/1(flag) -> Digital Write/1
  Chart/2(DesiredRate) -> Cast To Single5/1
  Subsystem1/1(xoor_interval) -> f_aoorInterval/1
  Cast To Single/1 -> Chart/3(activity_magnitude)
  Cast To Single1/1 -> Chart/4(MSR)
  Cast To Single2/1 -> Chart/5(LowerRateLimit)
  Cast To Single3/1 -> Chart/6(ResponseFactor)
  Cast To Single4/1 -> Chart/7(ActivityThreshold)
  Cast To Single5/1 -> xxir_ppm/1
  ReactionTime/1 -> Cast To Single7/1, Reaction_Time/1
  Cast To Single8/1 -> Chart/1(RecoveryTime)
  Cast To Single7/1 -> Chart/2(ReactionTime)
  Chart/3(CR) -> Cast To Single6/1, Cast To Single9/1, Current_Rate/1, AV Calculation/4(current_HR), Subsystem1/1(TargetRate)
  Cast To Single9/1 -> 1.1.2.3 WatchdogTimerForPulseDetection/10(XXIR_PPM)
  1.1.2.3 WatchdogTimerForPulseDetection/5(total_AAIR_rate_time) -> Output/1
  Subsystem/1(Out1) -> Cast To Single4/1, 1.1.2.4 CalculateUnsensedPace/5(AThresh)
  atrial_amp_Re/1 -> Atr_Amp_Reg/1
  vent_amp_Re/1 -> Vent_Amp_Reg/1
  dynAVDelay/1 -> AV Calculation/5(dyn_AV_delay), dyn_AV_delay/1
  fixedAVdelay/1 -> Cast To Single12/1, 1.1.2.3 WatchdogTimerForPulseDetection/13(AV_delay), fixed_AV_delay/1
  p_v_a_r_p_ext/1 -> PVARP_exten/1
  sensedAVDelayOffset/1 -> Cast To Single11/1, sensed_AV_offset/1
  ATR_dur/1 -> ATR_DUR/1
  ATR_fallback/1 -> ATR_FALL/1
  ATR_mode/1 -> ATR_MODE/1
  vent_blanking/1 -> ventBlanking/1
  min_AVdelay/1 -> Cast To Single10/1, min_AV_delay/1
  Subtract/1 -> Hdiff/1
  AV Calculation/1(AV_delay) -> AV_Delay/1
  Cast To Single10/1 -> AV Calculation/2(min_AV)
  Cast To Single11/1 -> AV Calculation/3(AV_offset)
  Cast To Single12/1 -> AV Calculation/1(fixed_AV)

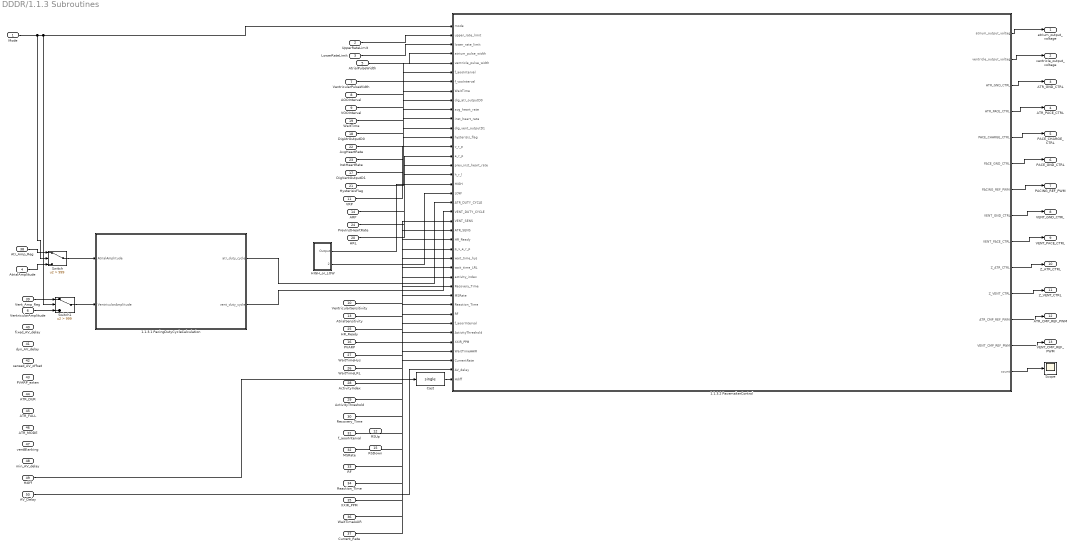
== system DDDR/1.1.3 Subroutines ==
  Mode : Inport
  UpperRateLimit : Inport  Port=2
  LowerRateLimit : Inport  Port=3
  AtrialAmplitude : Inport  Port=4
  AtrialPulseWidth : Inport  Port=5  OutDataTypeStr=double
  VentricularAmplitude : Inport  Port=6
  VentricularPulseWidth : Inport  Port=7  OutDataTypeStr=double
  AOOInterval : Inport  Port=8
  VOOInterval : Inport  Port=9
  VentricularSensitivity : Inport  Port=10
  VRP : Inport  Port=11
  RSUp : Inport  Port=12
  AtrialSensitivity : Inport  Port=13
  ARP : Inport  Port=14
  RSDown : Inport  Port=15
  PVARP : Inport  Port=16
  DigVentOutputD1 : Inport  Port=17
  DigAtrOutputD0 : Inport  Port=18
  WaitTime : Inport  Port=19
  HRL : Inport  Port=20
  HysterisisFlag : Inport  Port=21
  AvgHeartRate : Inport  Port=22
  InstHeartRate : Inport  Port=23
  PrevInstHeartRate : Inport  Port=24
  HR_Ready : Inport  Port=25
  WaitTimeLRL : Inport  Port=26
  WaitTimeHys : Inport  Port=27
  ActivityIndex : Inport  Port=28
  ActivityThreshold : Inport  Port=29
  Recovery_Time : Inport  Port=30
  f_aoorInterval : Inport  Port=31
  MSRate : Inport  Port=32
  RF : Inport  Port=33
  Reaction_Time : Inport  Port=34
  XXIR_PPM : Inport  Port=35
  WaitTimeAAIR : Inport  Port=36
  Current_Rate : Inport  Port=37
  Atr_Amp_Reg : Inport  Port=38
  Vent_Amp_Reg : Inport  Port=39
  fixed_AV_delay : Inport  Port=40
  dyn_AV_delay : Inport  Port=41
  sensed_AV_offset : Inport  Port=42
  PVARP_exten : Inport  Port=43
  ATR_DUR : Inport  Port=44
  ATR_FALL : Inport  Port=45
  ATR_MODE : Inport  Port=46
  ventBlanking : Inport  Port=47
  min_AV_delay : Inport  Port=48
  Hdiff : Inport  Port=49
  AV_Delay : Inport  Port=50
  1.1.3.1 PacingDutyCycleCalculation : Subsystem
  1.1.3.2 PacemakerControl : Stateflow chart  TreatAsAtomicUnit=on
      settings: PortSchema="{\"entries\":[{\"content\":{\"sides\":[{\"content\":{\"connectorIds\":[\"In1\",\"In2\",\"In3\",\"In4\",\"In5\",\"In6\",\"In7\",\"In8\",\"In12\",\"In10\",\"In11\",\"In9\",\"In13\",\"In14\",\"In15\",\"In16\",\"In17\",\"In18\",\"In19\",\"In20\",\"In21\",\"In22\",\"In23\",\"In24\",\"In25\",\"In26\",\"In27\",\"In28\",\"In29\",\"In30\",\"In31\",\"In32\",\"In33\",\"In34\",\"In35\",\"In36\",\"In37\",\"In38\",\"In39\"]},\"type\":\"ConnectorPlacement.EquallySpacedRectSide\",\"uuid\":\"d7a0a1d4-1adb-4f49-9409-b65f2a410999\"},{\"content\":{\"connectorIds\":[\"Out1\",\"Out2\",\"Out3\",\"Out4\",\"Out5\",\"Out6\",\"Out7\",\"Out8\",\"Out9\",\"Out10\",\"Out11\",\"Out12\",\"Out13\",\"Out14\"],\"side\":\"RIGHT\"},\"type\":\"ConnectorPlacement.EquallySpacedRectSide\",\"uuid\":\"f178eaad-70cd-4ec4-a78d-12af1cfbe493\"},{\"content\":{\"connectorIds\":[],\"side\":\"TOP\"},\"type\":\"ConnectorPlacement.EquallySpacedRectSide\",\"uuid\":\"df2c6513-3872-482b-abe5-5bf3da958119\"}]},\"type\":\"ConnectorPlacement.EquallySpacedConnector\",\"uuid\":\"0d6dffcb-0af9-47c5-9cde-377e88cba9d4\"}],\"packageUris\":[\"http://schema.mathworks.com/mf0/Connector/19700101\"],\"version\":\"1.0\"}"
  Cast : DataTypeConversion  OutDataTypeStr=single
  HIGH_or_LOW : Subsystem
      settings: PortSchema="{\"entries\":[{\"content\":{\"sides\":[{\"content\":{},\"type\":\"ConnectorPlacement.EquallySpacedRectSide\",\"uuid\":\"49d8c1b3-c71d-4c5e-9f29-3a8fe0514842\"},{\"content\":{\"side\":\"RIGHT\"},\"type\":\"ConnectorPlacement.EquallySpacedRectSide\",\"uuid\":\"0963f443-37bf-457e-bfcb-1d561403e5a9\"},{\"content\":{\"connectorIds\":[\"Out1\",\"Out2\"],\"side\":\"TOP\"},\"type\":\"ConnectorPlacement.EquallySpacedRectSide\",\"uuid\":\"32b78edd-16d0-4f55-b401-e4c12abc873e\"}]},\"type\":\"ConnectorPlacement.EquallySpacedConnector\",\"uuid\":\"974eb872-d95b-4224-a0e6-f13ce9826807\"}],\"packageUris\":[\"http://schema.mathworks.com/mf0/Connector/R2020b\"],\"version\":\"1.0\"}"
  Scope : Scope
  Switch : Switch  Criteria=u2 > Threshold  Threshold=999
  Switch1 : Switch  Criteria=u2 > Threshold  Threshold=999
  atrium_output_voltage : Outport
  ventricle_output_voltage : Outport  Port=2
  ATR_GND_CTRL : Outport  Port=3
  ATR_PACE_CTRL : Outport  Port=4
  PACE_CHARGE_CTRL : Outport  Port=5
  PACE_GND_CTRL : Outport  Port=6
  PACING_REF_PWM : Outport  Port=7
  VENT_GND_CTRL : Outport  Port=8
  VENT_PACE_CTRL : Outport  Port=9
  Z_ATR_CTRL : Outport  Port=10
  Z_VENT_CTRL : Outport  Port=11
  ATR_CMP_REF_PWM : Outport  Port=12
  VENT_CMP_REF_PWM : Outport  Port=13
  wires:
  Mode/1 -> Switch1/2, 1.1.3.2 PacemakerControl/1(mode), Switch/2
  1.1.3.2 PacemakerControl/1(atrium_output_voltage) -> atrium_output_voltage/1
  1.1.3.2 PacemakerControl/2(ventricle_output_voltage) -> ventricle_output_voltage/1
  UpperRateLimit/1 -> 1.1.3.2 PacemakerControl/2(upper_rate_limit)
  LowerRateLimit/1 -> 1.1.3.2 PacemakerControl/3(lower_rate_limit)
  AtrialPulseWidth/1 -> 1.1.3.2 PacemakerControl/4(atrium_pulse_width)
  VentricularPulseWidth/1 -> 1.1.3.2 PacemakerControl/5(ventricle_pulse_width)
  AOOInterval/1 -> 1.1.3.2 PacemakerControl/6(f_aooInterval)
  VOOInterval/1 -> 1.1.3.2 PacemakerControl/7(f_vooInterval)
  WaitTime/1 -> 1.1.3.2 PacemakerControl/8(WaitTime)
  DigVentOutputD1/1 -> 1.1.3.2 PacemakerControl/9(dig_vent_outputD1)
  DigAtrOutputD0/1 -> 1.1.3.2 PacemakerControl/12(dig_atr_outputD0)
  AvgHeartRate/1 -> 1.1.3.2 PacemakerControl/10(avg_heart_rate)
  InstHeartRate/1 -> 1.1.3.2 PacemakerControl/11(inst_heart_rate)
  HysterisisFlag/1 -> 1.1.3.2 PacemakerControl/13(hysterisis_flag)
  VRP/1 -> 1.1.3.2 PacemakerControl/14(v_r_p)
  ARP/1 -> 1.1.3.2 PacemakerControl/15(a_r_p)
  PrevInstHeartRate/1 -> 1.1.3.2 PacemakerControl/16(prev_inst_heart_rate)
  HRL/1 -> 1.1.3.2 PacemakerControl/17(h_r_l)
  HIGH_or_LOW/1(Output) -> 1.1.3.2 PacemakerControl/18(HIGH)
  HIGH_or_LOW/2(Output1) -> 1.1.3.2 PacemakerControl/19(LOW)
  1.1.3.2 PacemakerControl/11(Z_VENT_CTRL) -> Z_VENT_CTRL/1
  1.1.3.2 PacemakerControl/10(Z_ATR_CTRL) -> Z_ATR_CTRL/1
  1.1.3.2 PacemakerControl/9(VENT_PACE_CTRL) -> VENT_PACE_CTRL/1
  1.1.3.2 PacemakerControl/8(VENT_GND_CTRL) -> VENT_GND_CTRL/1
  1.1.3.2 PacemakerControl/7(PACING_REF_PWM) -> PACING_REF_PWM/1
  1.1.3.2 PacemakerControl/6(PACE_GND_CTRL) -> PACE_GND_CTRL/1
  1.1.3.2 PacemakerControl/3(ATR_GND_CTRL) -> ATR_GND_CTRL/1
  1.1.3.2 PacemakerControl/4(ATR_PACE_CTRL) -> ATR_PACE_CTRL/1
  1.1.3.2 PacemakerControl/5(PACE_CHARGE_CTRL) -> PACE_CHARGE_CTRL/1
  VentricularSensitivity/1 -> 1.1.3.2 PacemakerControl/22(VENT_SENS)
  AtrialSensitivity/1 -> 1.1.3.2 PacemakerControl/23(ATR_SENS)
  1.1.3.2 PacemakerControl/12(ATR_CMP_REF_PWM) -> ATR_CMP_REF_PWM/1
  1.1.3.2 PacemakerControl/13(VENT_CMP_REF_PWM) -> VENT_CMP_REF_PWM/1
  HR_Ready/1 -> 1.1.3.2 PacemakerControl/24(HR_Ready)
  1.1.3.2 PacemakerControl/14(count) -> Scope/1
  PVARP/1 -> 1.1.3.2 PacemakerControl/25(p_v_a_r_p)
  WaitTimeLRL/1 -> 1.1.3.2 PacemakerControl/27(wait_time_LRL)
  WaitTimeHys/1 -> 1.1.3.2 PacemakerControl/26(wait_time_hys)
  1.1.3.1 PacingDutyCycleCalculation/1(atr_duty_cycle) -> 1.1.3.2 PacemakerControl/20(ATR_DUTY_CYCLE)
  1.1.3.1 PacingDutyCycleCalculation/2(vent_duty_cycle) -> 1.1.3.2 PacemakerControl/21(VENT_DUTY_CYCLE)
  ActivityIndex/1 -> 1.1.3.2 PacemakerControl/28(activity_index)
  ActivityThreshold/1 -> 1.1.3.2 PacemakerControl/34(ActivityThreshold)
  Recovery_Time/1 -> 1.1.3.2 PacemakerControl/29(Recovery_Time)
  f_aoorInterval/1 -> 1.1.3.2 PacemakerControl/33(f_aoorInterval)
  MSRate/1 -> 1.1.3.2 PacemakerControl/30(MSRate)
  RF/1 -> 1.1.3.2 PacemakerControl/32(RF)
  Reaction_Time/1 -> 1.1.3.2 PacemakerControl/31(Reaction_Time)
  XXIR_PPM/1 -> 1.1.3.2 PacemakerControl/35(XXIR_PPM)
  WaitTimeAAIR/1 -> 1.1.3.2 PacemakerControl/36(WaitTimeAAIR)
  Current_Rate/1 -> 1.1.3.2 PacemakerControl/37(CurrentRate)
  AtrialAmplitude/1 -> Switch/3
  Atr_Amp_Reg/1 -> Switch/1
  Switch/1 -> 1.1.3.1 PacingDutyCycleCalculation/1(AtrialAmplitude)
  Vent_Amp_Reg/1 -> Switch1/1
  VentricularAmplitude/1 -> Switch1/3
  Switch1/1 -> 1.1.3.1 PacingDutyCycleCalculation/2(VentricularAmplitude)
  Hdiff/1 -> Cast/1
  Cast/1 -> 1.1.3.2 PacemakerControl/39(Hdiff)
  AV_Delay/1 -> 1.1.3.2 PacemakerControl/38(AV_delay)

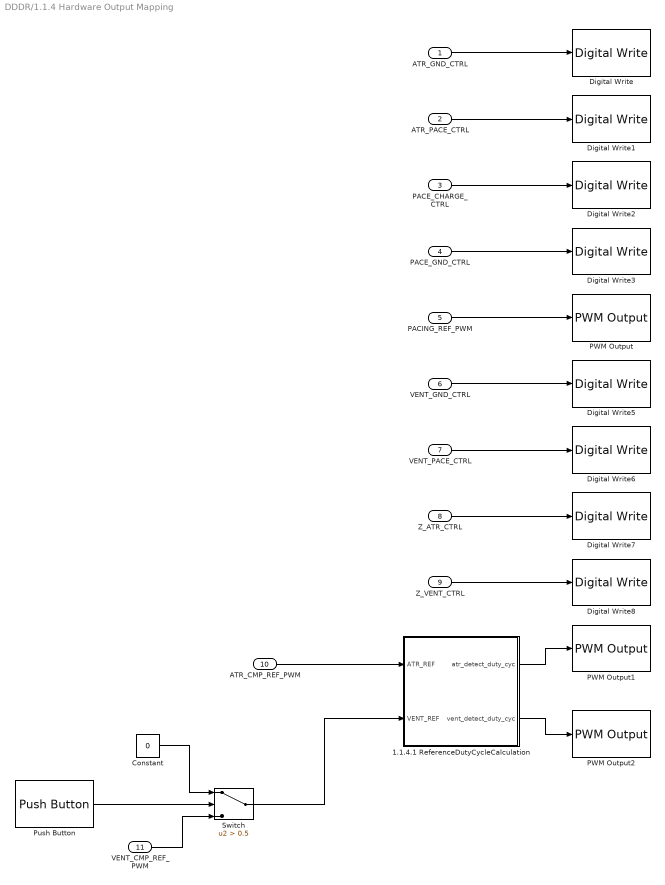
== system DDDR/1.1.4 Hardware Output Mapping ==
  ATR_GND_CTRL : Inport
  ATR_PACE_CTRL : Inport  Port=2
  PACE_CHARGE_CTRL : Inport  Port=3
  PACE_GND_CTRL : Inport  Port=4
  PACING_REF_PWM : Inport  Port=5
  VENT_GND_CTRL : Inport  Port=6
  VENT_PACE_CTRL : Inport  Port=7
  Z_ATR_CTRL : Inport  Port=8
  Z_VENT_CTRL : Inport  Port=9
  ATR_CMP_REF_PWM : Inport  Port=10
  VENT_CMP_REF_PWM : Inport  Port=11
  1.1.4.1 ReferenceDutyCycleCalculation : Subsystem
  Constant : Constant  Value=0
  Digital Write : frdmk64flib/Digital Write  Whichpin=PTD2 (D11)
  Digital Write1 : frdmk64flib/Digital Write  Whichpin=PTA0 (D8)
  Digital Write2 : frdmk64flib/Digital Write  Whichpin=PTB9 (D2)
  Digital Write3 : frdmk64flib/Digital Write  Whichpin=PTD0 (D10)
  Digital Write5 : frdmk64flib/Digital Write  Whichpin=PTD3 (D12)
  Digital Write6 : frdmk64flib/Digital Write  Whichpin=PTC4 (D9)
  Digital Write7 : frdmk64flib/Digital Write  Whichpin=PTB23 (D4)
  Digital Write8 : frdmk64flib/Digital Write  Whichpin=PTC3 (D7)
  PWM Output : frdmk64flib/PWM Output  Whichpin=PTA2 (D5)  InitialFrequency=2000  InitialDutyCycle=100
  PWM Output1 : frdmk64flib/PWM Output  Whichpin=PTC2 (D6)  InitialFrequency=2000  InitialDutyCycle=20
  PWM Output2 : frdmk64flib/PWM Output  Whichpin=PTA1 (D3)  InitialFrequency=2000  InitialDutyCycle=20
  Push Button : frdmk64flib/Push Button  Whichswitch=SW3  SampleTime1=-1
  Switch : Switch  Criteria=u2 > Threshold  Threshold=0.5
  wires:
  ATR_GND_CTRL/1 -> Digital Write/1
  ATR_PACE_CTRL/1 -> Digital Write1/1
  PACE_CHARGE_CTRL/1 -> Digital Write2/1
  PACE_GND_CTRL/1 -> Digital Write3/1
  VENT_GND_CTRL/1 -> Digital Write5/1
  VENT_PACE_CTRL/1 -> Digital Write6/1
  Z_ATR_CTRL/1 -> Digital Write7/1
  Z_VENT_CTRL/1 -> Digital Write8/1
  PACING_REF_PWM/1 -> PWM Output/1
  ATR_CMP_REF_PWM/1 -> 1.1.4.1 ReferenceDutyCycleCalculation/1(ATR_REF)
  VENT_CMP_REF_PWM/1 -> Switch/3
  1.1.4.1 ReferenceDutyCycleCalculation/1(atr_detect_duty_cyc) -> PWM Output1/1
  1.1.4.1 ReferenceDutyCycleCalculation/2(vent_detect_duty_cyc) -> PWM Output2/1
  Constant/1 -> Switch/1
  Switch/1 -> 1.1.4.1 ReferenceDutyCycleCalculation/2(VENT_REF)
  Push Button/1 -> Switch/2

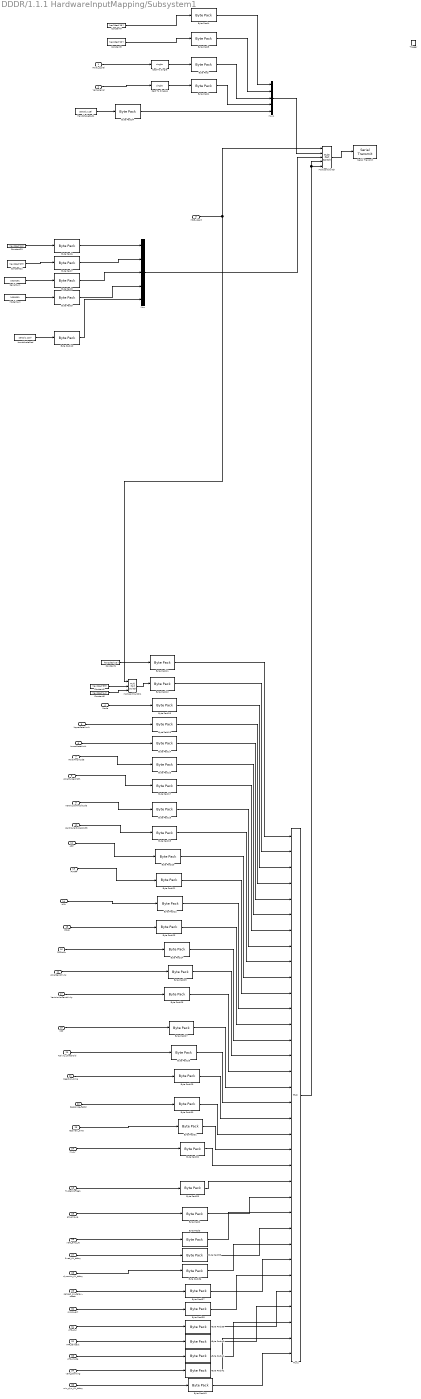
== system DDDR/1.1.1 HardwareInputMapping/Subsystem1 ==
  Atrial_signal : Inport
  Vent_signal : Inport  Port=2
  MSG_ident : Inport  Port=3  OutDataTypeStr=uint8
  Mode : Inport  Port=4
  UpperRateLimit : Inport  Port=5
  LowerRateLimit : Inport  Port=6  OutDataTypeStr=uint32
  AtrialAmplitude : Inport  Port=7
  AtrialPulseWidth : Inport  Port=8
  VentricularAmplitude : Inport  Port=9
  VentricularPulseWidth : Inport  Port=10
  AtrialSensitivity : Inport  Port=11
  ARP : Inport  Port=12
  PVARP : Inport  Port=13
  HRL : Inport  Port=14
  RSUp : Inport  Port=15
  RSDown : Inport  Port=16
  VentricularSensitivity : Inport  Port=17
  HysterisisFlag1 : Inport  Port=18
  VRP : Inport  Port=19
  Activity_threshold : Inport  Port=20
  Reaction_time : Inport  Port=21
  Response_factor : Inport  Port=22
  recovery_time : Inport  Port=23
  m_s_r : Inport  Port=24
  atr_amp_re : Inport  Port=25  OutDataTypeStr=single
  vent_amp_re : Inport  Port=26  OutDataTypeStr=single
  fixed_AV_delay : Inport  Port=27  OutDataTypeStr=uint32
  dynamic_AV_delay : Inport  Port=28  OutDataTypeStr=uint8
  sensed_AV_delay_offset : Inport  Port=29  OutDataTypeStr=int8
  pvarp_ext : Inport  Port=30  OutDataTypeStr=uint32
  ATR_dur : Inport  Port=31  OutDataTypeStr=uint32
  ATR_fallback : Inport  Port=32  OutDataTypeStr=uint8
  ATR_mode : Inport  Port=33  OutDataTypeStr=uint8
  vent_blanking : Inport  Port=34  OutDataTypeStr=uint8
  min_dyn_AV_delay : Inport  Port=35  OutDataTypeStr=uint8
  Trigger : TriggerPort  VariantControl=Variant  PortDimensions=1
  Byte Pack{,1..3,16,18,25..26} (8 alike) : etargetslib/Byte Pack  datatypes={'single'}  byteAlign=1
  Byte Pack{4..7,10..12,33..34,36,40..43} (14 alike) : etargetslib/Byte Pack  datatypes={'uint8'}  byteAlign=1
  Byte Pack{8..9,13..15,20..22,27..32,35,38..39} (17 alike) : etargetslib/Byte Pack  datatypes={'uint32'}  byteAlign=1
  Byte Pack{17,19,23..24} (4 alike) : etargetslib/Byte Pack  datatypes={'double'}  byteAlign=1
  Byte Pack37 : etargetslib/Byte Pack  datatypes={'int8'}  byteAlign=1
  Cast To Single : DataTypeConversion  OutDataTypeStr=single
  Cast To Single1 : DataTypeConversion  OutDataTypeStr=single
  Constant1 : Constant  Value=hex2dec('16')  OutDataTypeStr=uint8
  Constant2 : Constant  Value=hex2dec('39')  OutDataTypeStr=uint8
  Constant22 : Constant  Value=hex2dec('29')  OutDataTypeStr=uint8
  Constant23 : Constant  Value=hex2dec('16')  OutDataTypeStr=uint8
  Constant3 : Constant  Value=hex2dec('20')  OutDataTypeStr=uint8
  Constant4 : Constant  Value=hex2dec('16')  OutDataTypeStr=uint8
  Constant5 : Constant  Value=hex2dec('44')  OutDataTypeStr=uint8
  HandshakePad : Constant  Value=zeros(1,115)  OutDataTypeStr=uint8
  HandshakePad1 : Constant  Value=zeros(1,115)  OutDataTypeStr=uint8
  ModelNum : Constant  Value=1000001  OutDataTypeStr=uint32
  Multiport Switch : MultiPortSwitch  DataPortOrder=Zero-based contiguous  Inputs=4  zeroidx=on
  Multiport Switch1 : MultiPortSwitch  DataPortOrder=Specify indices  Inputs=2  DataPortIndices={2,3}
  Mux : Mux  Inputs=5
  Mux1 : Mux  Inputs=5
  Mux2 : Mux  Inputs=34
  Serial Transmit : frdmk64flib/Serial Transmit  SCIModule=0  Baudrate=uint32(9600)  Parity=None  StopBits=1  HardwareFlowControl=None  ByteOrder=LittleEndian  BlockingMode=on  OutputStatus=off
  SerialNum : Constant  Value=1010101  OutDataTypeStr=uint32
  wires:
  Byte Pack9/1 -> Mux/4
  ModelNum/1 -> Byte Pack9/1
  Byte Pack8/1 -> Mux/3
  Constant22/1 -> Byte Pack7/1
  Byte Pack10/1 -> Mux/5
  Constant23/1 -> Byte Pack6/1
  HandshakePad/1 -> Byte Pack10/1
  Byte Pack6/1 -> Mux/1
  Byte Pack7/1 -> Mux/2
  Byte Pack4/1 -> Mux1/1
  Cast To Single/1 -> Byte Pack/1
  Byte Pack1/1 -> Mux1/4
  Cast To Single1/1 -> Byte Pack1/1
  Constant4/1 -> Byte Pack4/1
  Byte Pack/1 -> Mux1/3
  Byte Pack5/1 -> Mux1/2
  Constant3/1 -> Byte Pack5/1
  Atrial_signal/1 -> Cast To Single/1
  Vent_signal/1 -> Cast To Single1/1
  Mux1/1 -> Multiport Switch/2
  SerialNum/1 -> Byte Pack8/1
  Mux/1 -> Multiport Switch/3
  Multiport Switch/1 -> Serial Transmit/1
  Constant1/1 -> Byte Pack11/1
  Mode/1 -> Byte Pack15/1
  UpperRateLimit/1 -> Byte Pack13/1
  LowerRateLimit/1 -> Byte Pack14/1
  AtrialAmplitude/1 -> Byte Pack16/1
  AtrialPulseWidth/1 -> Byte Pack17/1
  VentricularAmplitude/1 -> Byte Pack18/1
  VentricularPulseWidth/1 -> Byte Pack19/1
  ARP/1 -> Byte Pack20/1
  PVARP/1 -> Byte Pack21/1
  HRL/1 -> Byte Pack22/1
  RSUp/1 -> Byte Pack23/1
  RSDown/1 -> Byte Pack24/1
  AtrialSensitivity/1 -> Byte Pack25/1
  VentricularSensitivity/1 -> Byte Pack26/1
  VRP/1 -> Byte Pack27/1
  Activity_threshold/1 -> Byte Pack28/1
  Reaction_time/1 -> Byte Pack29/1
  Response_factor/1 -> Byte Pack30/1
  recovery_time/1 -> Byte Pack31/1
  m_s_r/1 -> Byte Pack32/1
  HysterisisFlag1/1 -> Byte Pack33/1
  Byte Pack11/1 -> Mux2/1
  Byte Pack12/1 -> Mux2/2
  Byte Pack15/1 -> Mux2/3
  Byte Pack13/1 -> Mux2/4
  Byte Pack14/1 -> Mux2/5
  Byte Pack16/1 -> Mux2/6
  Byte Pack17/1 -> Mux2/7
  Byte Pack18/1 -> Mux2/8
  Byte Pack19/1 -> Mux2/9
  Byte Pack20/1 -> Mux2/10
  Byte Pack21/1 -> Mux2/11
  Byte Pack22/1 -> Mux2/12
  Byte Pack23/1 -> Mux2/13
  Byte Pack24/1 -> Mux2/14
  Byte Pack25/1 -> Mux2/15
  Byte Pack26/1 -> Mux2/16
  Byte Pack27/1 -> Mux2/17
  Byte Pack28/1 -> Mux2/18
  Byte Pack29/1 -> Mux2/19
  Byte Pack30/1 -> Mux2/20
  Byte Pack31/1 -> Mux2/21
  Byte Pack32/1 -> Mux2/22
  Byte Pack33/1 -> Mux2/23
  Mux2/1 -> Multiport Switch/5, Multiport Switch/4
  Byte Pack34/1 -> Mux1/5
  HandshakePad1/1 -> Byte Pack34/1
  Constant2/1 -> Multiport Switch1/2
  Constant5/1 -> Multiport Switch1/3
  Multiport Switch1/1 -> Byte Pack12/1
  MSG_ident/1 -> Multiport Switch1/1, Multiport Switch/1
  atr_amp_re/1 -> Byte Pack2/1
  vent_amp_re/1 -> Byte Pack3/1
  fixed_AV_delay/1 -> Byte Pack35/1
  dynamic_AV_delay/1 -> Byte Pack36/1
  sensed_AV_delay_offset/1 -> Byte Pack37/1
  pvarp_ext/1 -> Byte Pack38/1
  ATR_dur/1 -> Byte Pack39/1
  ATR_fallback/1 -> Byte Pack40/1
  ATR_mode/1 -> Byte Pack41/1
  vent_blanking/1 -> Byte Pack42/1
  min_dyn_AV_delay/1 -> Byte Pack43/1
  Byte Pack2/1 -> Mux2/24
  Byte Pack3/1 -> Mux2/25
  Byte Pack35/1 -> Mux2/26
  Byte Pack36/1 -> Mux2/27
  Byte Pack37/1 -> Mux2/28
  Byte Pack38/1 -> Mux2/29
  Byte Pack39/1 -> Mux2/30
  Byte Pack40/1 -> Mux2/31
  Byte Pack41/1 -> Mux2/32
  Byte Pack42/1 -> Mux2/33
  Byte Pack43/1 -> Mux2/34

== system DDDR/1.1.1 HardwareInputMapping/Triggered Subsystem ==
  Trigger : TriggerPort  VariantControl=Variant
  FXOS8700 6-Axes Sensor : frdmk64flib/FXOS8700 6-Axes Sensor  Activesensor=Accelerometer only  ODR=800Hz  HybridODR=400Hz  Accelfullrange=-4g to +4g  SampleTime=-1
  Moving Average : dspstat3/Moving Average  Method=Sliding window  ForgettingFactorPort=off  SpecifyWindowLength=on  WindowLength=20  ForgettingFactor=0.9  SimulateUsing=Code generation
  Subsystem : Subsystem
  activity_magnitude : Outport
  wires:
  FXOS8700 6-Axes Sensor/1 -> Subsystem/1(In1)
  Subsystem/1(Output) -> Moving Average/1
  Moving Average/1 -> activity_magnitude/1

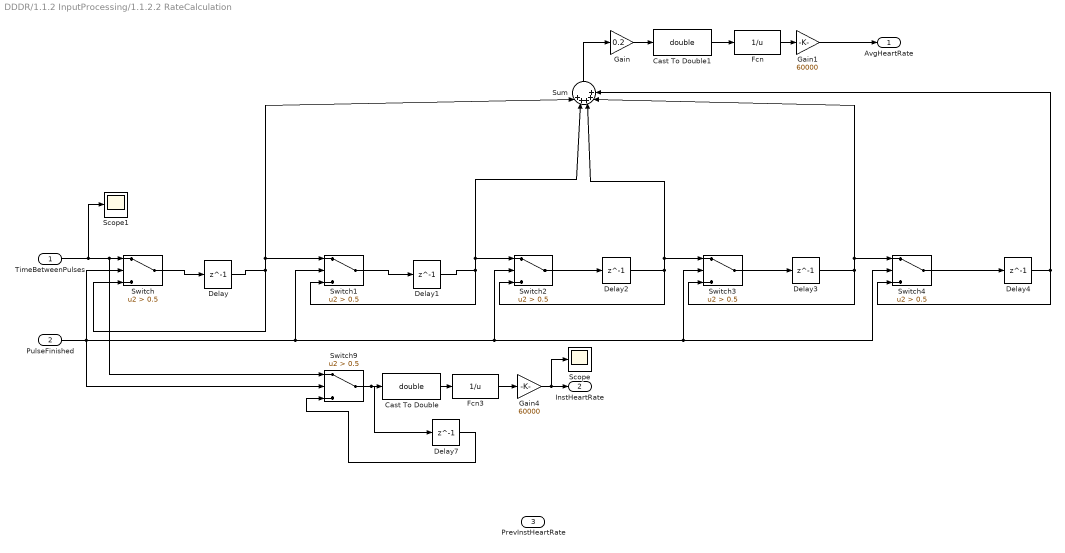
== system DDDR/1.1.2 InputProcessing/1.1.2.2 RateCalculation ==
  TimeBetweenPulses : Inport  OutDataTypeStr=uint32
  PulseFinished : Inport  Port=2  OutDataTypeStr=boolean
  Cast To Double : DataTypeConversion  OutDataTypeStr=double
  Cast To Double1 : DataTypeConversion  OutDataTypeStr=double
  Delay{,1..4} (5 alike) : Delay  DelayLength=1
  Delay7 : Delay  DelayLength=1  InitialCondition=0  SampleTime=0.001
  Fcn : Fcn  Expr=1/u
  Fcn3 : Fcn  Expr=1/u
  Gain : Gain  Gain=0.2
  Gain1 : Gain  Gain=60000
  Gain4 : Gain  Gain=60000
  Scope : Scope
  Scope1 : Scope
  Sum : Sum  Inputs=|+++++
  Switch{,1..4,9} (6 alike) : Switch  Criteria=u2 > Threshold  Threshold=0.5
  AvgHeartRate : Outport  OutDataTypeStr=double
  InstHeartRate : Outport  Port=2  OutDataTypeStr=double
  PrevInstHeartRate : Outport  Port=3  OutDataTypeStr=double
  wires:
  Fcn/1 -> Gain1/1
  Gain4/1 -> Scope/1, InstHeartRate/1
  Fcn3/1 -> Gain4/1
  Switch/1 -> Delay/1
  PulseFinished/1 -> Switch4/2, Switch3/2, Switch2/2, Switch1/2, Switch9/2, Switch/2
  Delay1/1 -> Sum/2, Switch2/1, Switch1/3
  TimeBetweenPulses/1 -> Switch9/1, Switch/1, Scope1/1
  Delay/1 -> Sum/1, Switch1/1, Switch/3
  Sum/1 -> Gain/1
  Switch4/1 -> Delay4/1
  Switch2/1 -> Delay2/1
  Delay2/1 -> Sum/3, Switch3/1, Switch2/3
  Switch3/1 -> Delay3/1
  Delay4/1 -> Sum/5, Switch4/3
  Delay3/1 -> Sum/4, Switch4/1, Switch3/3
  Gain1/1 -> AvgHeartRate/1
  Switch1/1 -> Delay1/1
  Switch9/1 -> Delay7/1, Cast To Double/1
  Delay7/1 -> Switch9/3
  Cast To Double/1 -> Fcn3/1
  Gain/1 -> Cast To Double1/1
  Cast To Double1/1 -> Fcn/1

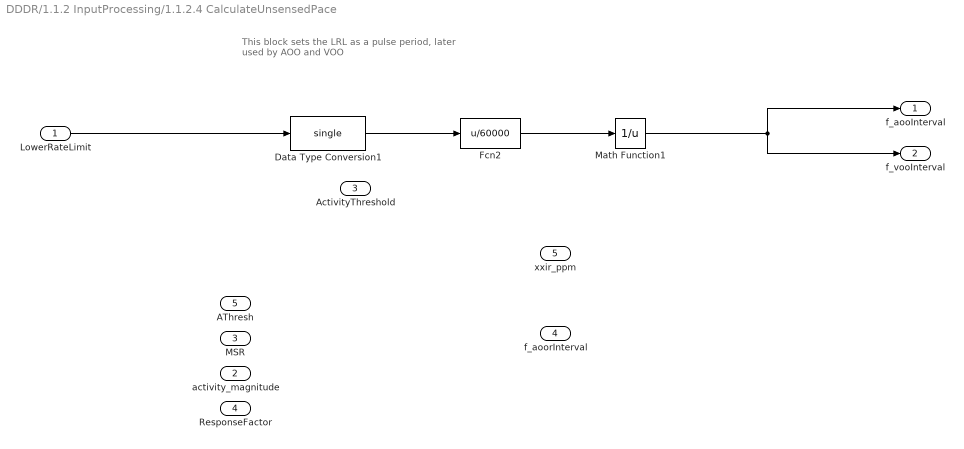
== system DDDR/1.1.2 InputProcessing/1.1.2.4 CalculateUnsensedPace ==
  note: This block sets the LRL as a pulse period, later
      | used by AOO and VOO
  LowerRateLimit : Inport
  activity_magnitude : Inport  Port=2
  MSR : Inport  Port=3
  ResponseFactor : Inport  Port=4
  AThresh : Inport  Port=5
  Data Type Conversion1 : DataTypeConversion  OutDataTypeStr=single
  Fcn2 : Fcn  Expr=u/60000
  Math Function1 : Math  Operator=reciprocal  SaturateOnIntegerOverflow=on
  f_aooInterval : Outport
  f_vooInterval : Outport  Port=2
  ActivityThreshold : Outport  Port=3
  f_aoorInterval : Outport  Port=4
  xxir_ppm : Outport  Port=5
  wires:
  Math Function1/1 -> f_vooInterval/1, f_aooInterval/1
  Data Type Conversion1/1 -> Fcn2/1
  Fcn2/1 -> Math Function1/1
  LowerRateLimit/1 -> Data Type Conversion1/1

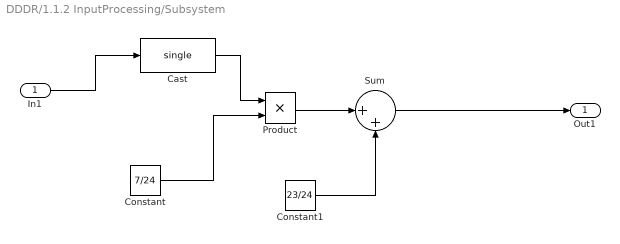
== system DDDR/1.1.2 InputProcessing/Subsystem ==
  In1 : Inport
  Cast : DataTypeConversion  OutDataTypeStr=single
  Constant : Constant  Value=7/24
  Constant1 : Constant  Value=23/24
  Product : Product
  Sum : Sum  Inputs=|++
  Out1 : Outport
  wires:
  Constant/1 -> Product/2
  Constant1/1 -> Sum/2
  Product/1 -> Sum/1
  Sum/1 -> Out1/1
  In1/1 -> Cast/1
  Cast/1 -> Product/1

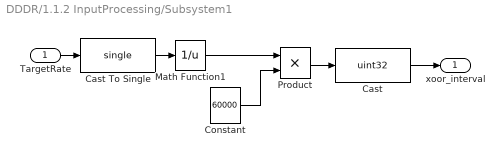
== system DDDR/1.1.2 InputProcessing/Subsystem1 ==
  TargetRate : Inport  OutDataTypeStr=single
  Cast : DataTypeConversion  OutDataTypeStr=uint32
  Cast To Single : DataTypeConversion  OutDataTypeStr=single
  Constant : Constant  Value=60000
  Math Function1 : Math  Operator=reciprocal  SaturateOnIntegerOverflow=on
  Product : Product
  xoor_interval : Outport  OutDataTypeStr=uint32
  wires:
  Constant/1 -> Product/2
  Math Function1/1 -> Product/1
  Product/1 -> Cast/1
  Cast/1 -> xoor_interval/1
  TargetRate/1 -> Cast To Single/1
  Cast To Single/1 -> Math Function1/1

== system DDDR/1.1.3 Subroutines/1.1.3.1 PacingDutyCycleCalculation ==
  AtrialAmplitude : Inport
  VentricularAmplitude : Inport  Port=2
  1.1.3.1.1 ATR Duty Cycle Calculation : Subsystem
  1.1.3.1.2 VENT Duty Cycle Calculation : Subsystem
  MaxVoltage : Constant  Value=5
  atr_duty_cycle : Outport
  vent_duty_cycle : Outport  Port=2
  wires:
  MaxVoltage/1 -> 1.1.3.1.2 VENT Duty Cycle Calculation/1(Input), 1.1.3.1.1 ATR Duty Cycle Calculation/2(In2)
  AtrialAmplitude/1 -> 1.1.3.1.1 ATR Duty Cycle Calculation/1(AtrialAmplitude)
  VentricularAmplitude/1 -> 1.1.3.1.2 VENT Duty Cycle Calculation/2(Input1)
  1.1.3.1.1 ATR Duty Cycle Calculation/1(Out1) -> atr_duty_cycle/1
  1.1.3.1.2 VENT Duty Cycle Calculation/1(Output) -> vent_duty_cycle/1

== system DDDR/1.1.3 Subroutines/HIGH_or_LOW ==
  HIGH : Constant  Value=true
  LOW : Constant  Value=false
  Output : Outport
  Output1 : Outport  Port=2
  wires:
  LOW/1 -> Output1/1
  HIGH/1 -> Output/1

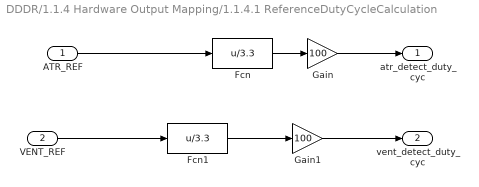
== system DDDR/1.1.4 Hardware Output Mapping/1.1.4.1 ReferenceDutyCycleCalculation ==
  ATR_REF : Inport
  VENT_REF : Inport  Port=2
  Fcn : Fcn  Expr=u/3.3
  Fcn1 : Fcn  Expr=u/3.3
  Gain : Gain  Gain=100
  Gain1 : Gain  Gain=100
  atr_detect_duty_cyc : Outport
  vent_detect_duty_cyc : Outport  Port=2
  wires:
  Fcn/1 -> Gain/1
  VENT_REF/1 -> Fcn1/1
  Gain/1 -> atr_detect_duty_cyc/1
  Fcn1/1 -> Gain1/1
  Gain1/1 -> vent_detect_duty_cyc/1
  ATR_REF/1 -> Fcn/1
